simulink model "General_Model"  (R2023b)
settings: Solver=FixedStepDiscrete  StartTime=0.0  StopTime=runtime  FixedStep=Ts  RelTol=1e-3  EnableMultiTasking=on
InitFcn:
  | Ts=1; % Time Step
  | runtime = 3600*5.5;%14400
StopFcn:
  | plotResults = true ;% turn off if unwanted
  | 
  | if plotResults
  | 
  | out = out_BattModel.BatteryValidationScope;
  | 
  | % Get Signals from simulation output.
  | time = out.time;
  | TestSignal = out.signals.values(:,1);
  | SOC = out.signals.values(:,2);
  | BattPower = out.signals.values(:,3);
  | EnergyThrough = out.signals.values(:,4);
  | EnergyLost = out.signals.values(:,5);
  | 
  | %% Create Figure
  | fig_Validation_Results = figure;
  | 
  | % X-axis
  | step = 3600;
  | myxtick = 0:step:time(end);
  | myxticklabel = 0:time(end)/step ;
  | 
  | % TestSignal
  | subplot(4,1,1);
  | hold on;
  | plot(time, TestSignal, '-', 'LineWidth', 2,'Color','black');
  | xticks(myxtick);
  | xticklabels(myxticklabel);
  | xlabel('Time (hours)');
  | ylim 'padded'
  | ylabel('Power (kW)');
  | %legend('TestSignal', 'Location', 'northwest');
  | title('Test Signal');
  | grid on;
  | box on
  | 
  | % BattPower
  | subplot(4,1,3);
  | stairs(time, BattPower, 'LineWidth', 2,'Color',	"#D95319"); % Orange
  | yticks([-4 -2 0 2 4 6 ]);
  | xticks(myxtick);
  | xticklabels(myxticklabel);
  | xlabel('Time (hours)');
  | ylim 'padded'
  | ylabel('Power [kW]');
  | %legend('BattPower','Location', 'northwest')
  | title('Battery Power');
  | grid on;
  | box on
  | 
  | % SOC
  | subplot(4,1,2);
  | plot(time, SOC, '-', 'LineWidth', 3);
  | xticks(myxtick);
  | xticklabels(myxticklabel);
  | xlabel('Time (hours)');
  | yticks(0:20:100);
  | ylim 'padded'
  | ylabel('SOC in %');
  | %yline(battery_min_soc,'--','LineWidth', 1.5)
  | %yline(battery_max_soc,'--','LineWidth', 1.5)
  | %str = sprintf('Battery (%dkWh)',battery_capacity);
  | %legend(str, 'Location', 'northwest');
  | title('Battery State of Charge (SOC)');
  | grid on;
  | box on
  | 
  | % Energy
  | subplot(4,1,4);
  | hold on
  | plot(time, EnergyThrough,'-', 'LineWidth', 2)
  | plot(time, EnergyLost,'-', 'LineWidth', 2)
  | xticks(myxtick);
  | xticklabels(myxticklabel);
  | xlabel('Time (hours)');
  | ylim 'padded'
  | ylabel('Power (kW)');
  | legend( 'Energy Through','Energy Lost','Location', 'northwest');%, 'Location', 'northeast', 'Orientation', 'vertical', 'Position', [0.75, 0.2, 0.05, 0.05]);
  | title('Energy Through and Energy Lost');
  | grid on;
  | box on
  | 
  | % Stretch Figure
  | figwidth = 8; % Width in inches
  | figheight = 8; % Height in inches
  | set(gcf, 'Units', 'Inches', 'Position', [1, 1, figwidth, figheight]);
  | 
  | % Save Files
  | saveas(fig_Validation_Results, 'BatteryValidation_Results', 'epsc')
  | saveas(fig_Validation_Results, 'BatteryValidation_Results', 'pdf')
  | 
  | disp('\nFigures saved as PDF and eps')
  | 
  | 
  | 
  | 
  | 
  | end
undefined symbols (not defined in the file): DiscIntNeverNeededParam, sigbuilder_block
libraries: spspowerguiLib x1
settings Model: Creator=mas  LastModifiedBy=leons
settings SolverCC: AlgebraicLoopSolver=TrustRegion
settings DataIOCC: LimitDataPoints=on  SaveFormat=Array  SignalLoggingSaveFormat=ModelDataLogs  SaveTime=off  ReturnWorkspaceOutputsName=out_BattModel
settings OptimizationCC: ExpressionDepthLimit=2147483647  LifeSpan=inf
settings DebuggingCC: UnderspecifiedInitializationDetection=Classic  MergeDetectMultiDrivingBlocksExec=none  SolverPrmCheckMsg=warning  FcnCallInpInsideContextMsg=warning  UnconnectedInputMsg=warning  UnconnectedOutputMsg=warning  UnconnectedLineMsg=warning  StateNameClashWarn=warning  SFUnexpectedBacktrackingDiag=warning  SFNoUnconditionalDefaultTransitionDiag=warning  SFExecutionAtInitializationDiag=none  ArithmeticOperatorsInVariantConditions=warning
settings HardwareCC: ProdBitPerPointer=32  ProdBitPerSizeT=32  ProdBitPerPtrDiffT=32  ProdLargestAtomicFloat=None  ProdIntDivRoundTo=Undefined  ProdEndianess=Unspecified  ProdWordSize=32  ProdHWDeviceType=32-bit Generic
settings ModelReferenceCC: EnableRefExpFcnMdlSchedulingChecks=on  PropagateSignalLabelsOutOfModel=off
settings SFSimCC: SimUseLocalCustomCode=off  CustomCodeUndefinedFunction=UseInterfaceOnly
settings RTWCC: RTWUseLocalCustomCode=off  DLArmComputeVersion=19.05
settings CodeAppCC: StateflowObjectComments=on
settings GRTTargetCC: TargetLangStandard=C89/C90 (ANSI)  CombineOutputUpdateFcns=off  GRTInterface=on
settings ConfigComp: CovMetricSettings=dw  CovSaveCumulativeToWorkspaceVar=on  CovSaveSingleToWorkspaceVar=on  CovExternalEMLEnable=off  CovSFcnEnable=off

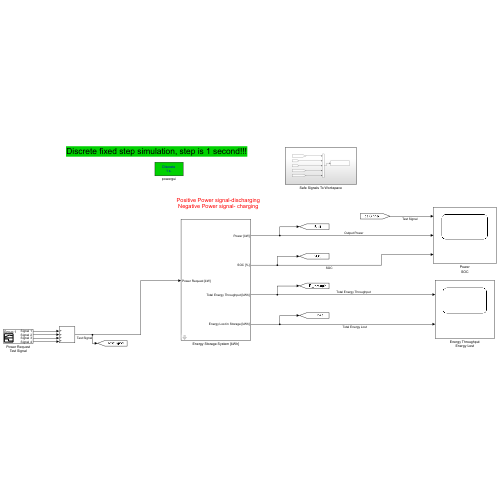
[thumbnail: Simulink's stored preview of the top-level diagram]
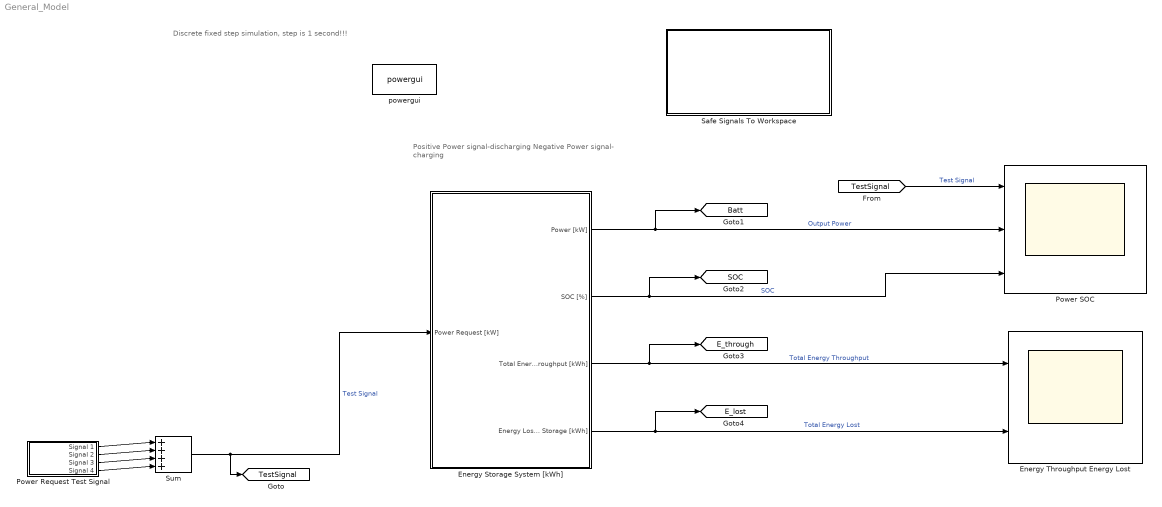
== system General_Model ==
  note: Discrete fixed step simulation, step is 1 second!!!
  note: Positive Power signal-discharging
      | Negative Power signal- charging
  Energy Storage System [kWh] : Subsystem  mask{Pmax=5, Emax=10, SOCinit=25, Eff=95, SOCmax=100, SOCmin=20, second=1}
      mask prompts: Pmax "Max Power [kW] (both for charging and discharging)"; Emax "Total Storage Energy [kWh]"; SOCinit "Initial SOC [%]"; Eff "Round Trip Efficiency [%]"; SOCmax "SOC max [%]"; SOCmin "SOC min [%]"; second "Seconds to Runtime relation (= 1 if runtime in seconds; = 1/60 if runtime in minutes; = 1/3600 if runtime in hours)"
  Energy Throughput Energy Lost : Scope  NumInputPorts=2
  Power SOC : Scope  NumInputPorts=3
  Power Request Test Signal : Subsystem  Tag=STV Subsys  LoadFcn=sigbuilder_block('load');  StartFcn=sigbuilder_block('start');  StopFcn=sigbuilder_block('stop');  ClipboardFcn=sigbuilder_block('clipboard');  mask(Sigbuilder block){tuvar=[0:10]}
      mask help: Simulink:masks:SigbuilderBlock_MD
      mask init:
      | if ~strcmp(get_param(bdroot(gcbh),'SimulationStatus'),'stopped') tuvar = sigbuilder_block('maskInit'); end
      settings: CopyFcn=sigbuilder_block('copy');  DeleteFcn=sigbuilder_block('delete');  ModelCloseFcn=sigbuilder_block('modelClose');  PreSaveFcn=sigbuilder_block('preSave');  PauseFcn=sigbuilder_block('pause');  ContinueFcn=sigbuilder_block('continue');  NameChangeFcn=sigbuilder_block('namechange');  OpenFcn=sigbuilder_block('open',[768.6 36.6 766.8 549.6 ]);  CloseFcn=sigbuilder_block('close');
      mask Display: plot(0, 0, 100, 100,[2, 2, 32, 32, 2], [68, 8, 8, 68, 68],[32, 2], [38, 38], [32, 19, 2],[53, 60, 44], [32, 17, 17, 2],[16, 16, 31, 31]);txt = getActiveGroup(gcbh);text(2, 100, txt,'verticalAlignment', 'top');
  Safe Signals To Workspace : Subsystem
  Sum : Sum  Inputs=|++++
  powergui : spspowerguiLib/powergui  Priority=1  SimulationMode=Discrete  SampleTime=1  frequency=60  Iterations=50  frequencyindice=60  Pbase=100e6  ErrMax=1e-4  UnitsV=kV  UnitsW=MW  buscounter=0  FunctionMessages=off  echomessages=off  EnableUseOfTLC=off  CurrentSourceSwitches=off  DisableSnubberDevices=off  DisableRonSwitches=off  DisableVfSwitches=off  DisplayEquations=off  AutomaticDiscreteSolvers=off  SolverType=Tustin/Backward Euler (TBE)  Interpol=off  ExternalGateDelay=off  methode=off  Ts=100  x0status=blocks  SPID=on  SwTol=0  HookPort=off  NonlinearTolerance=1e-4  nMaxIteration=100  ContinueOnMaxIteration=off  RestoreLinks=warning  ResistiveCurrentMeasurement=off  Frange=[0:2:500]  Ylog=off  Xlog=on  ShowGrid=off  save=off  variable=ZData  structure=0  ZoomFFT=off  StartTime=0.0  cycles=1  DisplayStyle=1  fundamental=60  FreqAxis=off  MaxFrequency=1000  frequencyindicesteady=1  RmsSteady=1  display=off
  tag scope: Batt=global, E_lost=global, E_through=global, SOC=global, TestSignal=global
  wires:
  Power Request Test Signal/1(Signal 1) -> Sum/1
  Power Request Test Signal/3(Signal 3) -> Sum/3
  Power Request Test Signal/4(Signal 4) -> Sum/4
  Power Request Test Signal/2(Signal 2) -> Sum/2
  Sum/1 -> Energy Storage System [kWh]/1(Power Request [kW]), [TestSignal]  "Test Signal"
  Energy Storage System [kWh]/2(SOC [%]) -> [SOC], Power SOC/3  "SOC"
  Energy Storage System [kWh]/4(" Energy Lost in Storage [kWh]") -> [E_lost], Energy Throughput Energy Lost/2  "Total Energy Lost"
  Energy Storage System [kWh]/3(Total Energy Throughput [kWh]) -> Energy Throughput Energy Lost/1, [E_through]  "Total Energy Throughput"
  Energy Storage System [kWh]/1(Power [kW]) -> Power SOC/2, [Batt]  "Output Power"
  [TestSignal] -> Power SOC/1  "Test Signal"

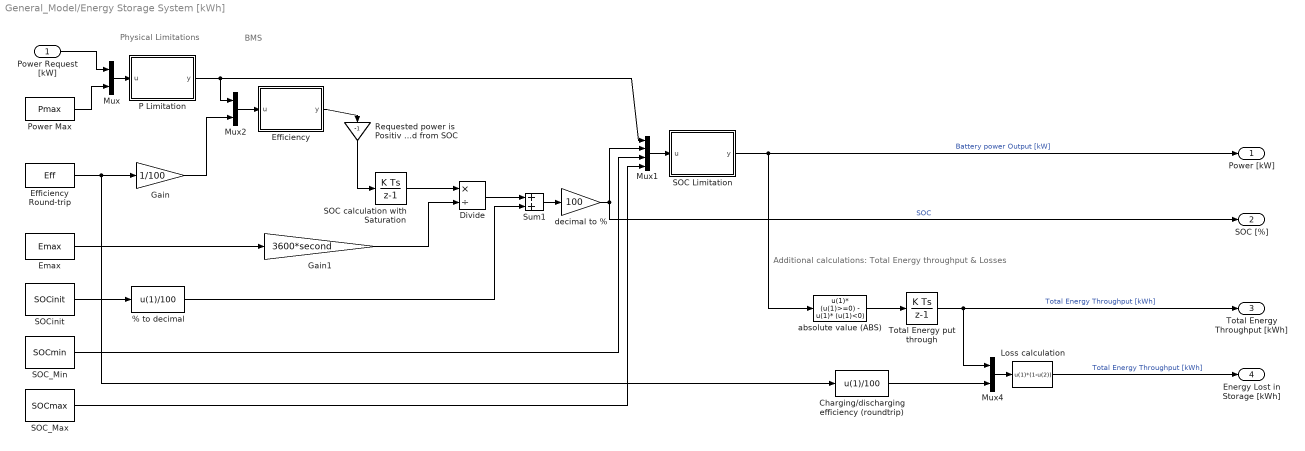
== system General_Model/Energy Storage System [kWh] ==
  note: Additional calculations: Total Energy throughput & Losses
  note: Physical Limitations
  note: BMS
  Power Request [kW] : Inport
  % to decimal : Fcn  Expr=u(1)/100
  Charging/discharging efficiency (roundtrip) : Fcn  Expr=u(1)/100
  Divide : Product  Inputs=*/
  Efficiency : MATLAB Function  TreatAsAtomicUnit=on
  Efficiency Round-trip : Constant  Value=Eff
  Emax : Constant  Value=Emax
  Gain : Gain  Gain=1/100
  Gain1 : Gain  Gain=3600*second
  Loss calculation : Fcn  Expr=u(1)*(1-u(2))
  Mux : Mux  Inputs=2
  Mux1 : Mux
  Mux2 : Mux  Inputs=2
  Mux4 : Mux  Inputs=2
  P Limitation : MATLAB Function  TreatAsAtomicUnit=on
  Power Max : Constant  Value=Pmax
  Requested power is Positiv but needs to be substracted from SOC : Gain  Gain=-1
  SOC Limitation : MATLAB Function  TreatAsAtomicUnit=on
  SOC calculation with Saturation : DiscreteIntegrator  gainval=1  SampleTime=Ts  LimitOutput=on  UpperSaturationLimit=(SOCmax/100 - SOCinit/100 ) * Emax*3600*second  LowerSaturationLimit=(+SOCmin/100 - SOCinit/100 ) *Emax*3600*second  ICPrevOutput=DiscIntNeverNeededParam  ICPrevScaledInput=DiscIntNeverNeededParam
  SOC_Max : Constant  Value=SOCmax
  SOC_Min : Constant  Value=SOCmin
  SOCinit : Constant  Value=SOCinit
  Sum1 : Sum
  Total Energy put through : DiscreteIntegrator  gainval=1/(3600*second)  SampleTime=Ts  ICPrevOutput=DiscIntNeverNeededParam  ICPrevScaledInput=DiscIntNeverNeededParam
  absolute value (ABS) : Fcn  Expr=u(1)* (u(1)>=0) - u(1)* (u(1)<0)
  decimal to % : Gain  Gain=100
  Power [kW] : Outport
  SOC [%] : Outport  Port=2
  Total Energy Throughput [kWh] : Outport  Port=3
  " Energy Lost in Storage [kWh]" : Outport  Port=4
  wires:
  Mux/1 -> P Limitation/1(u)
  decimal to %/1 -> Mux1/2, SOC [%]/1  "SOC"
  Efficiency Round-trip/1 -> Charging/discharging efficiency (roundtrip)/1, Gain/1
  SOCinit/1 -> % to decimal/1
  Sum1/1 -> decimal to %/1
  Divide/1 -> Sum1/1
  SOC calculation with Saturation/1 -> Divide/1
  % to decimal/1 -> Sum1/2
  Mux1/1 -> SOC Limitation/1(u)
  SOC Limitation/1(y) -> Power [kW]/1, absolute value (ABS)/1  "Battery power Output [kW]"
  Requested power is Positiv but needs to be substracted from SOC/1 -> SOC calculation with Saturation/1
  P Limitation/1(y) -> Mux2/1, Mux1/1
  Gain/1 -> Mux2/2
  Mux2/1 -> Efficiency/1(u)
  Total Energy put through/1 -> Mux4/1, Total Energy Throughput [kWh]/1  "Total Energy Throughput [kWh]"
  absolute value (ABS)/1 -> Total Energy put through/1
  Emax/1 -> Gain1/1
  Mux4/1 -> Loss calculation/1
  Loss calculation/1 -> " Energy Lost in Storage [kWh]"/1  "Total Energy Throughput [kWh]"
  SOC_Min/1 -> Mux1/3
  SOC_Max/1 -> Mux1/4
  Power Max/1 -> Mux/2
  Power Request [kW]/1 -> Mux/1
  Charging/discharging efficiency (roundtrip)/1 -> Mux4/2
  Efficiency/1(y) -> Requested power is Positiv but needs to be substracted from SOC/1
  Gain1/1 -> Divide/2

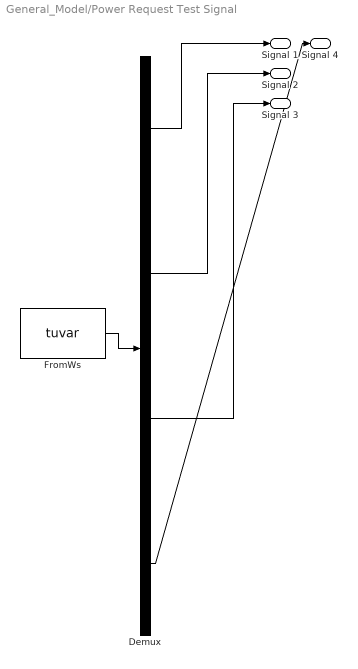
== system General_Model/Power Request Test Signal ==
  Demux : Demux  Tag=STV Demux
      settings: DisplayOption=none
  FromWs : FromWorkspace  Tag=STV FromWs  VariableName=tuvar
      SigBuilderData=|
      | common.afterFinalStr = 'Extrapolate'
      | common.sampleTime = 0
      | dataSet.timeRange = [0 25200]
      | dataSet.name = 'Group 1'
      | sbobj.Groups.Name = 'Group 1'
      | sbobj.Groups.Signals(1).Name = 'Signal 1'
      | sbobj.Groups.Signals(1).XData = [0 1 1 3600 3600 25200]
      | sbobj.Groups.Signals(1).YData = [0 0 1 1 0 0]
      | sbobj.Groups.Signals(2).Name = 'Signal 2'
      | sbobj.Groups.Signals(2).XData = [0 3601 3601 10800 10800 25200]
      | sbobj.Groups.Signals(2).YData = [0 -0.01 -4 -4 0 0]
      | sbobj.Groups.Signals(3).Name = 'Signal 3'
      | sbobj.Groups.Signals(3).XData = [0 12780 12780 18000 18000 25200]
      | sbobj.Groups.Signals(3).YData = [0 0 6 6 0 0]
      | sbobj.Groups.Signals(4).Name = 'Signal 4'
      | sbobj.Groups.Signals(4).XData = [0 18001 18001 21600 21600 25200]
      | sbobj.Groups.Signals(4).YData = [0 0 -6 -6 0 0]
      | sbobj.Groups.TimeRange = [0 25200]
  Signal 1 : Outport  Tag=STV Outport
  Signal 2 : Outport  Tag=STV Outport  Port=2
  Signal 3 : Outport  Tag=STV Outport  Port=3
  Signal 4 : Outport  Tag=STV Outport  Port=4
  wires:
  Demux/3 -> Signal 3/1
  Demux/2 -> Signal 2/1
  FromWs/1 -> Demux/1
  Demux/1 -> Signal 1/1
  Demux/4 -> Signal 4/1

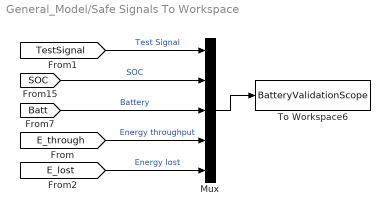
== system General_Model/Safe Signals To Workspace ==
  Mux : Mux  Inputs=5
  To Workspace6 : ToWorkspace  VariableName=BatteryValidationScope  SaveFormat=Structure With Time  SampleTime=-1
  wires:
  Mux/1 -> To Workspace6/1
  [SOC] -> Mux/2  "SOC"
  [TestSignal] -> Mux/1  "Test Signal"
  [Batt] -> Mux/3  "Battery"
  [E_through] -> Mux/4  "Energy throughput"
  [E_lost] -> Mux/5  "Energy lost"

== matlab function General_Model/Energy Storage System [kWh]/Efficiency ==
  data: u input; y output
function y = fcn(u)
Preq = u(1);
Roundtrip_eff = u(2) ;
eff = sqrt(Roundtrip_eff);

if ( Preq>0) % Discharging
    Power_stored = Preq/eff; % for Discharging Preq_new = Preq/eff
else % charging
    Power_stored = Preq*eff; % for Charging Preq_new = Preq*eff
end

y = Power_stored;

% If i request Power, due to losses i need to request more than i actaully
% need => Preq_new = Preq/eff
% If i want to charge the Battery, due to losses The acutally stored Power
% is smaller than what i put in
% => Preq_new = Preq*eff

== matlab function General_Model/Energy Storage System [kWh]/SOC Limitation ==
  data: u input; y output
function y = fcn(u)
Pout = u(1);
SOC = u(2) ;
SOC_min = u(3);
SOC_max = u(4);

if ( SOC<=SOC_min || SOC>=SOC_max)
    Pout = 0;
end

y = Pout;

== matlab function General_Model/Energy Storage System [kWh]/P Limitation ==
  data: u input; y output
function y = fcn(u)
y = min(max(u(1), -u(2)), u(2));
